simulink model "simulink_lab3"  (R2022b)
settings: Solver=VariableStepAuto  StartTime=0.0  StopTime=10.0  RelTol=1e-3
settings Model: Creator=DSP-27  LastModifiedBy=DSP-27

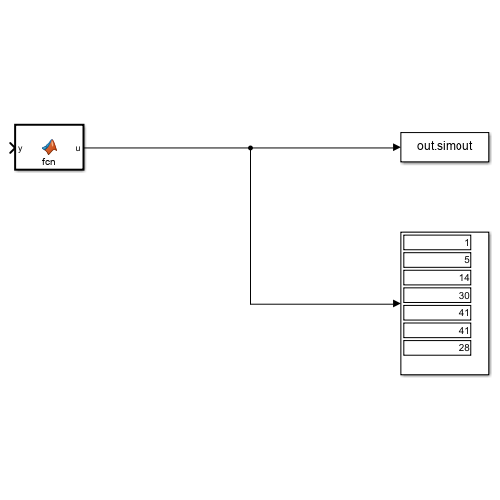
[thumbnail: Simulink's stored preview of the top-level diagram]
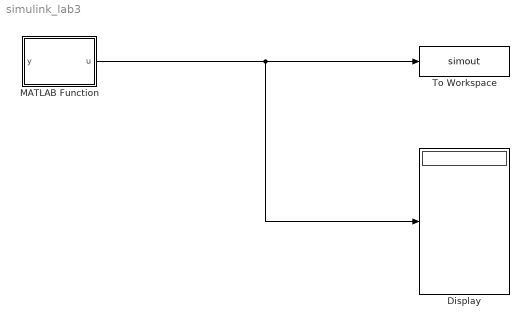
== system simulink_lab3 ==
  Display : Display
  MATLAB Function : MATLAB Function  TreatAsAtomicUnit=on
  To Workspace : ToWorkspace  VariableName=simout  SaveFormat=Timeseries  SampleTime=-1
  wires:
  MATLAB Function/1(u) -> Display/1, To Workspace/1

== matlab function simulink_lab3/MATLAB Function ==
  data: y input; u output
function u = fcn(y)

x = [1,2,3,4];
h = [1,3,5,7];
x1 = length(x);
h1 = length(h);
y = zeros(1,x1+h1-1);

for i = 1:x1
    for j = 1:h1
        y(i+j-1) = y(i+j-1)+x(i)*h(j);
    end
end

u = y;
